simulink library "cmc_command_and_mode_control"  (R2015a)
settings: Solver=ode45  StartTime=0.0  StopTime=10.0  RelTol=1e-3
undefined symbols (not defined in the file or in its folder): mlp_command_list, mlp_command_times, mlp_dummy_state_cmd, mlp_loc_mode_cmd_list, mlp_loc_mode_cmd_times, mlp_mode_cmd_list, mlp_mode_cmd_times, mlp_num_commands, mlp_num_mode_cmds, mlp_speed_gain_cmd_list, mlp_speed_gain_cmd_times
libraries: simulink x4
settings Model: Creator=rhnakamu  LastModifiedBy=rhnakamu

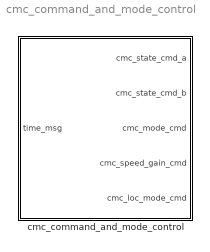
== system cmc_command_and_mode_control ==
  cmc_command_and_mode_control : Subsystem

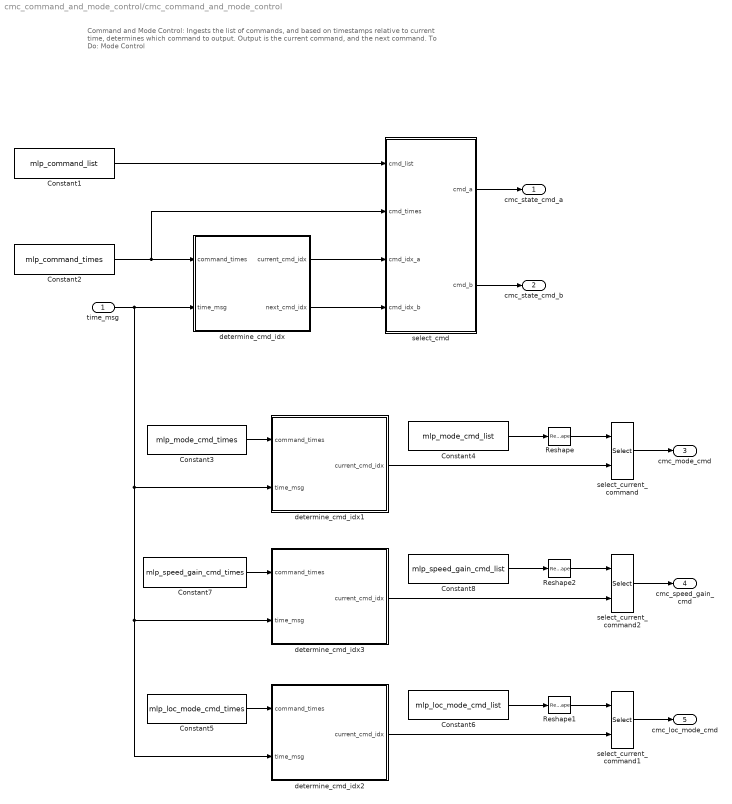
== system cmc_command_and_mode_control/cmc_command_and_mode_control ==
  note: Command and Mode Control:
      | 	Ingests the list of commands, and based on timestamps relative to current time, determines which command to output.
      | 	Output is the current command, and the next command.
      |
      | To Do:
      | 	Mode Control
  time_msg : Inport
  Constant1 : Constant  Value=mlp_command_list
  Constant2 : Constant  Value=mlp_command_times
  Constant3 : Constant  Value=mlp_mode_cmd_times
  Constant4 : Constant  Value=mlp_mode_cmd_list
  Constant5 : Constant  Value=mlp_loc_mode_cmd_times
  Constant6 : Constant  Value=mlp_loc_mode_cmd_list
  Constant7 : Constant  Value=mlp_speed_gain_cmd_times
  Constant8 : Constant  Value=mlp_speed_gain_cmd_list
  Reshape : Reshape  OutputDimensionality=Column vector (2-D)
  Reshape1 : Reshape  OutputDimensionality=Column vector (2-D)
  Reshape2 : Reshape  OutputDimensionality=Column vector (2-D)
  determine_cmd_idx : Subsystem
  determine_cmd_idx1 : Subsystem
  determine_cmd_idx2 : Subsystem
  determine_cmd_idx3 : Subsystem
  select_cmd : Subsystem
  select_current_command : Selector  NumberOfDimensions=2  InputPortWidth=3  IndexOptions=Index vector (port),Select all  Indices=[1 3],1  OutputSizes=1,1
  select_current_command1 : Selector  NumberOfDimensions=2  InputPortWidth=3  IndexOptions=Index vector (port),Select all  Indices=[1 3],1  OutputSizes=1,1
  select_current_command2 : Selector  NumberOfDimensions=2  InputPortWidth=3  IndexOptions=Index vector (port),Select all  Indices=[1 3],1  OutputSizes=1,1
  cmc_state_cmd_a : Outport  OutDataTypeStr=Bus: cmc_state_cmd
  cmc_state_cmd_b : Outport  Port=2  OutDataTypeStr=Bus: cmc_state_cmd
  cmc_mode_cmd : Outport  Port=3
  cmc_speed_gain_cmd : Outport  Port=4
  cmc_loc_mode_cmd : Outport  Port=5
  wires:
  Reshape2/1 -> select_current_command2/1
  Constant8/1 -> Reshape2/1
  determine_cmd_idx3/1(current_cmd_idx) -> select_current_command2/2
  Constant7/1 -> determine_cmd_idx3/1(command_times)
  select_current_command2/1 -> cmc_speed_gain_cmd/1
  Reshape1/1 -> select_current_command1/1
  Constant6/1 -> Reshape1/1
  determine_cmd_idx2/1(current_cmd_idx) -> select_current_command1/2
  Constant5/1 -> determine_cmd_idx2/1(command_times)
  select_current_command1/1 -> cmc_loc_mode_cmd/1
  time_msg/1 -> determine_cmd_idx/2(time_msg), determine_cmd_idx1/2(time_msg), determine_cmd_idx2/2(time_msg), determine_cmd_idx3/2(time_msg)
  Reshape/1 -> select_current_command/1
  Constant4/1 -> Reshape/1
  determine_cmd_idx1/1(current_cmd_idx) -> select_current_command/2
  Constant3/1 -> determine_cmd_idx1/1(command_times)
  select_current_command/1 -> cmc_mode_cmd/1
  Constant2/1 -> determine_cmd_idx/1(command_times), select_cmd/2(cmd_times)
  Constant1/1 -> select_cmd/1(cmd_list)
  select_cmd/2(cmd_b) -> cmc_state_cmd_b/1
  determine_cmd_idx/2(next_cmd_idx) -> select_cmd/4(cmd_idx_b)
  select_cmd/1(cmd_a) -> cmc_state_cmd_a/1
  determine_cmd_idx/1(current_cmd_idx) -> select_cmd/3(cmd_idx_a)

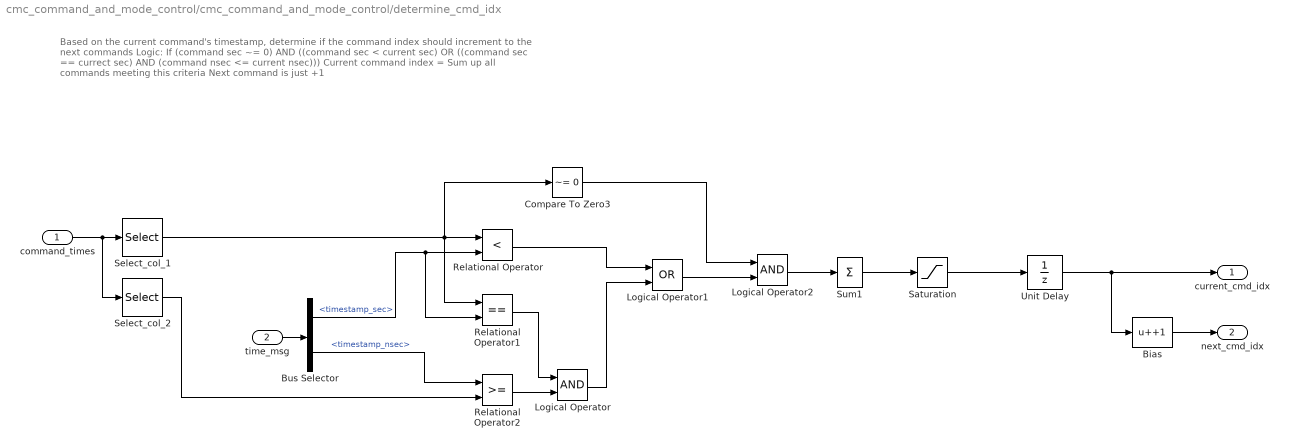
== system cmc_command_and_mode_control/cmc_command_and_mode_control/determine_cmd_idx ==
  note: Based on the current command's timestamp, determine if the command index should increment to the next commands
      |
      | Logic:
      | If (command sec ~= 0) AND ((command sec < current sec) OR ((command sec == currect sec) AND (command nsec <= current nsec)))
      | Current command index = Sum up all commands meeting this criteria
      | Next command is just +1
  command_times : Inport
  time_msg : Inport  Port=2
  Bias : Bias  Bias=+1
  Bus Selector : BusSelector  OutputSignals=timestamp_sec,timestamp_nsec
  Compare To Zero3 : simulink/Logic and Bit Operations/Compare To Zero  relop=~=  OutDataTypeStr=boolean
  Logical Operator : Logic  AllPortsSameDT=off  OutDataTypeStr=boolean
  Logical Operator1 : Logic  Operator=OR  AllPortsSameDT=off  OutDataTypeStr=boolean
  Logical Operator2 : Logic  AllPortsSameDT=off  OutDataTypeStr=boolean
  Relational Operator : RelationalOperator  Operator=<  OutDataTypeStr=boolean
  Relational Operator1 : RelationalOperator  Operator===  OutDataTypeStr=boolean
  Relational Operator2 : RelationalOperator  OutDataTypeStr=boolean
  Saturation : Saturate  UpperLimit=mlp_num_commands  LowerLimit=1
      settings: AttributesFormatString=|
      | UL: %<UpperLimit>
      | LL: %<LowerLimit>
  Select_col_1 : Selector  NumberOfDimensions=2  InputPortWidth=3  IndexOptions=Select all,Index vector (dialog)  Indices=[1 3],1  OutputSizes=1,1
  Select_col_2 : Selector  NumberOfDimensions=2  InputPortWidth=3  IndexOptions=Select all,Index vector (dialog)  Indices=[1 3],2  OutputSizes=1,1
  Sum1 : Sum  Inputs=+
  Unit Delay : UnitDelay  InitialCondition=1  SampleTime=-1
  current_cmd_idx : Outport
  next_cmd_idx : Outport  Port=2
  wires:
  Unit Delay/1 -> current_cmd_idx/1, Bias/1
  Saturation/1 -> Unit Delay/1
  Sum1/1 -> Saturation/1
  Bus Selector/2 -> Relational Operator2/1  "<timestamp_nsec>"
  Bus Selector/1 -> Relational Operator/2, Relational Operator1/2  "<timestamp_sec>"
  Select_col_2/1 -> Relational Operator2/2
  Select_col_1/1 -> Relational Operator/1, Relational Operator1/1, Compare To Zero3/1
  Relational Operator/1 -> Logical Operator1/1
  Logical Operator/1 -> Logical Operator1/2
  Relational Operator1/1 -> Logical Operator/1
  Relational Operator2/1 -> Logical Operator/2
  Bias/1 -> next_cmd_idx/1
  time_msg/1 -> Bus Selector/1
  Logical Operator2/1 -> Sum1/1
  Compare To Zero3/1 -> Logical Operator2/1
  Logical Operator1/1 -> Logical Operator2/2
  command_times/1 -> Select_col_1/1, Select_col_2/1

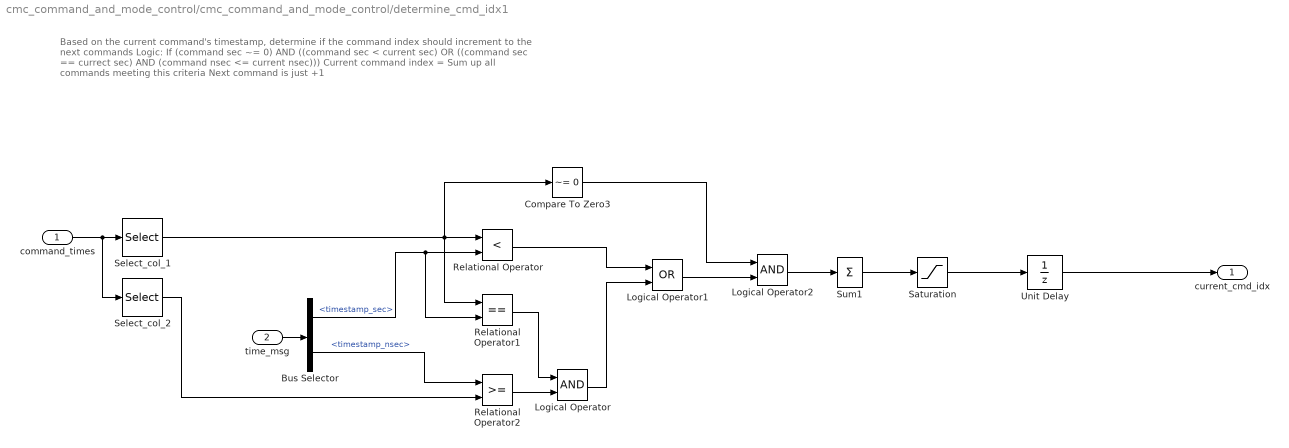
== system cmc_command_and_mode_control/cmc_command_and_mode_control/determine_cmd_idx1 ==
  note: Based on the current command's timestamp, determine if the command index should increment to the next commands
      |
      | Logic:
      | If (command sec ~= 0) AND ((command sec < current sec) OR ((command sec == currect sec) AND (command nsec <= current nsec)))
      | Current command index = Sum up all commands meeting this criteria
      | Next command is just +1
  command_times : Inport
  time_msg : Inport  Port=2
  Bus Selector : BusSelector  OutputSignals=timestamp_sec,timestamp_nsec
  Compare To Zero3 : simulink/Logic and Bit Operations/Compare To Zero  relop=~=  OutDataTypeStr=boolean
  Logical Operator : Logic  AllPortsSameDT=off  OutDataTypeStr=boolean
  Logical Operator1 : Logic  Operator=OR  AllPortsSameDT=off  OutDataTypeStr=boolean
  Logical Operator2 : Logic  AllPortsSameDT=off  OutDataTypeStr=boolean
  Relational Operator : RelationalOperator  Operator=<  OutDataTypeStr=boolean
  Relational Operator1 : RelationalOperator  Operator===  OutDataTypeStr=boolean
  Relational Operator2 : RelationalOperator  OutDataTypeStr=boolean
  Saturation : Saturate  UpperLimit=mlp_num_mode_cmds  LowerLimit=1
      settings: AttributesFormatString=|
      | UL: %<UpperLimit>
      | LL: %<LowerLimit>
  Select_col_1 : Selector  NumberOfDimensions=2  InputPortWidth=3  IndexOptions=Select all,Index vector (dialog)  Indices=[1 3],1  OutputSizes=1,1
  Select_col_2 : Selector  NumberOfDimensions=2  InputPortWidth=3  IndexOptions=Select all,Index vector (dialog)  Indices=[1 3],2  OutputSizes=1,1
  Sum1 : Sum  Inputs=+
  Unit Delay : UnitDelay  InitialCondition=1  SampleTime=-1
  current_cmd_idx : Outport
  wires:
  command_times/1 -> Select_col_2/1, Select_col_1/1
  Logical Operator1/1 -> Logical Operator2/2
  Compare To Zero3/1 -> Logical Operator2/1
  Logical Operator2/1 -> Sum1/1
  time_msg/1 -> Bus Selector/1
  Relational Operator2/1 -> Logical Operator/2
  Relational Operator1/1 -> Logical Operator/1
  Logical Operator/1 -> Logical Operator1/2
  Relational Operator/1 -> Logical Operator1/1
  Select_col_1/1 -> Compare To Zero3/1, Relational Operator1/1, Relational Operator/1
  Select_col_2/1 -> Relational Operator2/2
  Bus Selector/1 -> Relational Operator1/2, Relational Operator/2  "<timestamp_sec>"
  Bus Selector/2 -> Relational Operator2/1  "<timestamp_nsec>"
  Sum1/1 -> Saturation/1
  Saturation/1 -> Unit Delay/1
  Unit Delay/1 -> current_cmd_idx/1

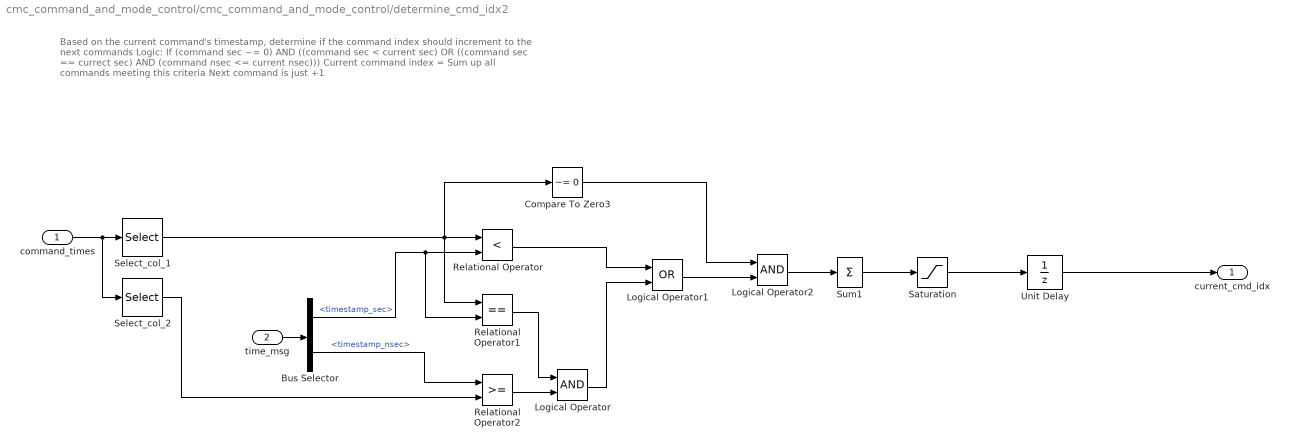
== system cmc_command_and_mode_control/cmc_command_and_mode_control/determine_cmd_idx2 ==
  note: Based on the current command's timestamp, determine if the command index should increment to the next commands
      |
      | Logic:
      | If (command sec ~= 0) AND ((command sec < current sec) OR ((command sec == currect sec) AND (command nsec <= current nsec)))
      | Current command index = Sum up all commands meeting this criteria
      | Next command is just +1
  command_times : Inport
  time_msg : Inport  Port=2
  Bus Selector : BusSelector  OutputSignals=timestamp_sec,timestamp_nsec
  Compare To Zero3 : simulink/Logic and Bit Operations/Compare To Zero  relop=~=  OutDataTypeStr=boolean
  Logical Operator : Logic  AllPortsSameDT=off  OutDataTypeStr=boolean
  Logical Operator1 : Logic  Operator=OR  AllPortsSameDT=off  OutDataTypeStr=boolean
  Logical Operator2 : Logic  AllPortsSameDT=off  OutDataTypeStr=boolean
  Relational Operator : RelationalOperator  Operator=<  OutDataTypeStr=boolean
  Relational Operator1 : RelationalOperator  Operator===  OutDataTypeStr=boolean
  Relational Operator2 : RelationalOperator  OutDataTypeStr=boolean
  Saturation : Saturate  UpperLimit=mlp_num_mode_cmds  LowerLimit=1
      settings: AttributesFormatString=|
      | UL: %<UpperLimit>
      | LL: %<LowerLimit>
  Select_col_1 : Selector  NumberOfDimensions=2  InputPortWidth=3  IndexOptions=Select all,Index vector (dialog)  Indices=[1 3],1  OutputSizes=1,1
  Select_col_2 : Selector  NumberOfDimensions=2  InputPortWidth=3  IndexOptions=Select all,Index vector (dialog)  Indices=[1 3],2  OutputSizes=1,1
  Sum1 : Sum  Inputs=+
  Unit Delay : UnitDelay  InitialCondition=1  SampleTime=-1
  current_cmd_idx : Outport
  wires:
  Unit Delay/1 -> current_cmd_idx/1
  Saturation/1 -> Unit Delay/1
  Sum1/1 -> Saturation/1
  Bus Selector/2 -> Relational Operator2/1  "<timestamp_nsec>"
  Bus Selector/1 -> Relational Operator/2, Relational Operator1/2  "<timestamp_sec>"
  Select_col_2/1 -> Relational Operator2/2
  Select_col_1/1 -> Relational Operator/1, Relational Operator1/1, Compare To Zero3/1
  Relational Operator/1 -> Logical Operator1/1
  Logical Operator/1 -> Logical Operator1/2
  Relational Operator1/1 -> Logical Operator/1
  Relational Operator2/1 -> Logical Operator/2
  time_msg/1 -> Bus Selector/1
  Logical Operator2/1 -> Sum1/1
  Compare To Zero3/1 -> Logical Operator2/1
  Logical Operator1/1 -> Logical Operator2/2
  command_times/1 -> Select_col_1/1, Select_col_2/1

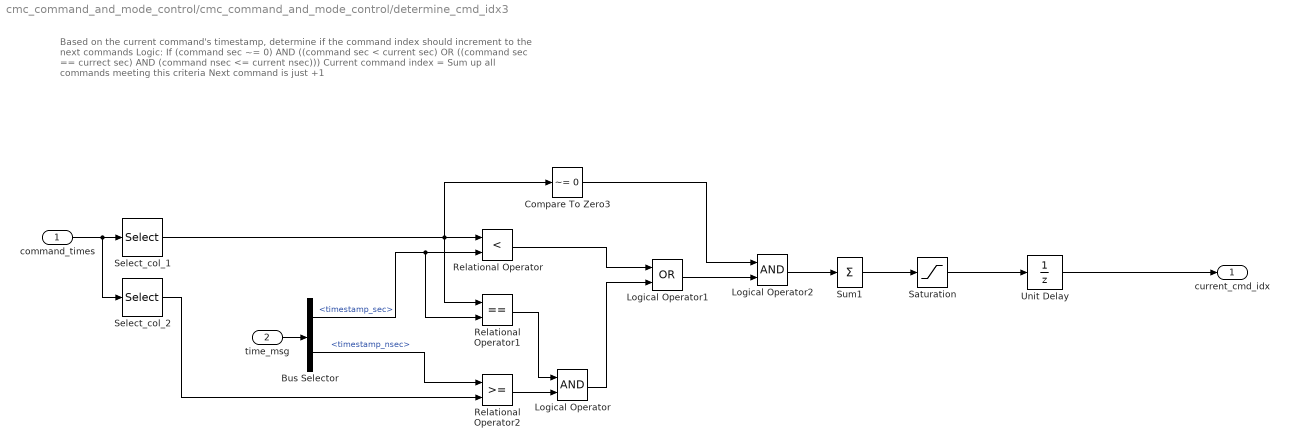
== system cmc_command_and_mode_control/cmc_command_and_mode_control/determine_cmd_idx3 ==
  note: Based on the current command's timestamp, determine if the command index should increment to the next commands
      |
      | Logic:
      | If (command sec ~= 0) AND ((command sec < current sec) OR ((command sec == currect sec) AND (command nsec <= current nsec)))
      | Current command index = Sum up all commands meeting this criteria
      | Next command is just +1
  command_times : Inport
  time_msg : Inport  Port=2
  Bus Selector : BusSelector  OutputSignals=timestamp_sec,timestamp_nsec
  Compare To Zero3 : simulink/Logic and Bit Operations/Compare To Zero  relop=~=  OutDataTypeStr=boolean
  Logical Operator : Logic  AllPortsSameDT=off  OutDataTypeStr=boolean
  Logical Operator1 : Logic  Operator=OR  AllPortsSameDT=off  OutDataTypeStr=boolean
  Logical Operator2 : Logic  AllPortsSameDT=off  OutDataTypeStr=boolean
  Relational Operator : RelationalOperator  Operator=<  OutDataTypeStr=boolean
  Relational Operator1 : RelationalOperator  Operator===  OutDataTypeStr=boolean
  Relational Operator2 : RelationalOperator  OutDataTypeStr=boolean
  Saturation : Saturate  UpperLimit=mlp_num_mode_cmds  LowerLimit=1
      settings: AttributesFormatString=|
      | UL: %<UpperLimit>
      | LL: %<LowerLimit>
  Select_col_1 : Selector  NumberOfDimensions=2  InputPortWidth=3  IndexOptions=Select all,Index vector (dialog)  Indices=[1 3],1  OutputSizes=1,1
  Select_col_2 : Selector  NumberOfDimensions=2  InputPortWidth=3  IndexOptions=Select all,Index vector (dialog)  Indices=[1 3],2  OutputSizes=1,1
  Sum1 : Sum  Inputs=+
  Unit Delay : UnitDelay  InitialCondition=1  SampleTime=-1
  current_cmd_idx : Outport
  wires:
  command_times/1 -> Select_col_2/1, Select_col_1/1
  Logical Operator1/1 -> Logical Operator2/2
  Compare To Zero3/1 -> Logical Operator2/1
  Logical Operator2/1 -> Sum1/1
  time_msg/1 -> Bus Selector/1
  Relational Operator2/1 -> Logical Operator/2
  Relational Operator1/1 -> Logical Operator/1
  Logical Operator/1 -> Logical Operator1/2
  Relational Operator/1 -> Logical Operator1/1
  Select_col_1/1 -> Compare To Zero3/1, Relational Operator1/1, Relational Operator/1
  Select_col_2/1 -> Relational Operator2/2
  Bus Selector/1 -> Relational Operator1/2, Relational Operator/2  "<timestamp_sec>"
  Bus Selector/2 -> Relational Operator2/1  "<timestamp_nsec>"
  Sum1/1 -> Saturation/1
  Saturation/1 -> Unit Delay/1
  Unit Delay/1 -> current_cmd_idx/1

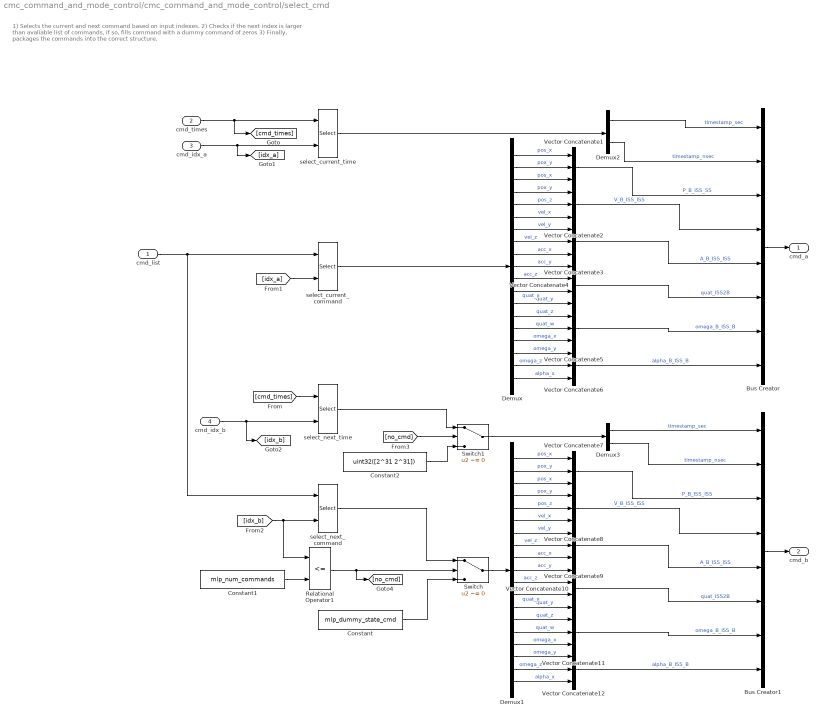
== system cmc_command_and_mode_control/cmc_command_and_mode_control/select_cmd ==
  note: 1) Selects the current and next command based on input indexes.
      | 2) Checks if the next index is larger than avaliable list of commands, if so, fills command with a dummy command of zeros
      | 3) Finally, packages the commands into the correct structure.
  cmd_list : Inport
  cmd_times : Inport  Port=2
  cmd_idx_a : Inport  Port=3
  cmd_idx_b : Inport  Port=4
  Bus Creator : BusCreator  Inputs=8  OutDataTypeStr=Bus: cmc_state_cmd
      settings: InheritFromInputs=off
  Bus Creator1 : BusCreator  Inputs=8  OutDataTypeStr=Bus: cmc_state_cmd
      settings: InheritFromInputs=off
  Constant : Constant  Value=mlp_dummy_state_cmd
  Constant1 : Constant  Value=mlp_num_commands
  Constant2 : Constant  Value=uint32([2^31 2^31])
  Demux : Demux  Outputs=19
  Demux1 : Demux  Outputs=19
  Demux2 : Demux  Outputs=2
  Demux3 : Demux  Outputs=2
  Relational Operator1 : RelationalOperator  Operator=<=  OutDataTypeStr=boolean
  Switch : Switch  Criteria=u2 ~= 0
  Switch1 : Switch  Criteria=u2 ~= 0
  Vector Concatenate{1..3,5..9,11..12} (10 alike) : Concatenate  NumInputs=3
  Vector Concatenate10 : Concatenate  NumInputs=4
  Vector Concatenate4 : Concatenate  NumInputs=4
  select_current_command : Selector  NumberOfDimensions=2  InputPortWidth=3  IndexOptions=Index vector (port),Select all  Indices=[1 3],1  OutputSizes=1,1
  select_current_time : Selector  NumberOfDimensions=2  InputPortWidth=3  IndexOptions=Index vector (port),Select all  Indices=[1 3],1  OutputSizes=1,1
  select_next_command : Selector  NumberOfDimensions=2  InputPortWidth=3  IndexOptions=Index vector (port),Select all  Indices=[1 3],1  OutputSizes=1,1
  select_next_time : Selector  NumberOfDimensions=2  InputPortWidth=3  IndexOptions=Index vector (port),Select all  Indices=[1 3],1  OutputSizes=1,1
  cmd_a : Outport
  cmd_b : Outport  Port=2
  wires:
  Constant2/1 -> Switch1/3
  [no_cmd] -> Switch1/2
  select_next_time/1 -> Switch1/1
  Switch1/1 -> Demux3/1
  [idx_b] -> select_next_command/2, Relational Operator1/1
  cmd_idx_b/1 -> select_next_time/2, [idx_b]
  [idx_a] -> select_current_command/2
  cmd_idx_a/1 -> select_current_time/2, [idx_a]
  [cmd_times] -> select_next_time/1
  select_current_time/1 -> Demux2/1
  cmd_times/1 -> select_current_time/1, [cmd_times]
  Demux1/19 -> Vector Concatenate12/3  "alpha_x"
  Demux1/18 -> Vector Concatenate12/2  "omega_z"
  Demux1/17 -> Vector Concatenate12/1  "omega_y"
  Demux1/16 -> Vector Concatenate11/3  "omega_x"
  Demux1/15 -> Vector Concatenate11/2  "quat_w"
  Demux1/14 -> Vector Concatenate11/1  "quat_z"
  Demux1/13 -> Vector Concatenate10/4  "quat_y"
  Demux1/12 -> Vector Concatenate10/3  "quat_x"
  Demux1/11 -> Vector Concatenate10/2  "acc_z"
  Demux1/10 -> Vector Concatenate10/1  "acc_y"
  Demux1/9 -> Vector Concatenate9/3  "acc_x"
  Demux1/8 -> Vector Concatenate9/2  "vel_z"
  Demux1/7 -> Vector Concatenate9/1  "vel_y"
  Demux1/6 -> Vector Concatenate8/3  "vel_x"
  Demux1/5 -> Vector Concatenate8/2  "pos_z"
  Demux1/4 -> Vector Concatenate8/1  "pox_y"
  Demux1/3 -> Vector Concatenate7/3  "pos_x"
  Demux1/2 -> Vector Concatenate7/2  "pox_y"
  Demux1/1 -> Vector Concatenate7/1  "pos_x"
  Vector Concatenate12/1 -> Bus Creator1/8  "alpha_B_ISS_B"
  Vector Concatenate11/1 -> Bus Creator1/7  "omega_B_ISS_B"
  Vector Concatenate10/1 -> Bus Creator1/6  "quat_ISS2B"
  Vector Concatenate9/1 -> Bus Creator1/5  "A_B_ISS_ISS"
  Vector Concatenate8/1 -> Bus Creator1/4  "V_B_ISS_ISS"
  Vector Concatenate7/1 -> Bus Creator1/3  "P_B_ISS_ISS"
  Switch/1 -> Demux1/1
  Demux/19 -> Vector Concatenate6/3  "alpha_x"
  Demux/18 -> Vector Concatenate6/2  "omega_z"
  Demux/17 -> Vector Concatenate6/1  "omega_y"
  Demux/16 -> Vector Concatenate5/3  "omega_x"
  Demux/15 -> Vector Concatenate5/2  "quat_w"
  Demux/14 -> Vector Concatenate5/1  "quat_z"
  Demux/13 -> Vector Concatenate4/4  "quat_y"
  Demux/12 -> Vector Concatenate4/3  "quat_x"
  Demux/11 -> Vector Concatenate4/2  "acc_z"
  Demux/10 -> Vector Concatenate4/1  "acc_y"
  Demux/9 -> Vector Concatenate3/3  "acc_x"
  Demux/8 -> Vector Concatenate3/2  "vel_z"
  Demux/7 -> Vector Concatenate3/1  "vel_y"
  Demux/6 -> Vector Concatenate2/3  "vel_x"
  Demux/5 -> Vector Concatenate2/2  "pos_z"
  Demux/4 -> Vector Concatenate2/1  "pox_y"
  Demux/3 -> Vector Concatenate1/3  "pos_x"
  Demux/2 -> Vector Concatenate1/2  "pox_y"
  Demux/1 -> Vector Concatenate1/1  "pos_x"
  Demux3/2 -> Bus Creator1/2  "timestamp_nsec"
  Demux3/1 -> Bus Creator1/1  "timestamp_sec"
  Bus Creator1/1 -> cmd_b/1
  Vector Concatenate6/1 -> Bus Creator/8  "alpha_B_ISS_B"
  Vector Concatenate5/1 -> Bus Creator/7  "omega_B_ISS_B"
  Vector Concatenate4/1 -> Bus Creator/6  "quat_ISS2B"
  Vector Concatenate3/1 -> Bus Creator/5  "A_B_ISS_ISS"
  Vector Concatenate2/1 -> Bus Creator/4  "V_B_ISS_ISS"
  Vector Concatenate1/1 -> Bus Creator/3  "P_B_ISS_SS"
  Demux2/2 -> Bus Creator/2  "timestamp_nsec"
  Demux2/1 -> Bus Creator/1  "timestamp_sec"
  cmd_list/1 -> select_current_command/1, select_next_command/1
  select_next_command/1 -> Switch/1
  Constant/1 -> Switch/3
  Constant1/1 -> Relational Operator1/2
  Relational Operator1/1 -> Switch/2, [no_cmd]
  select_current_command/1 -> Demux/1
  Bus Creator/1 -> cmd_a/1
